simulink model "Simulation"  (R2023b)
settings: Solver=VariableStepAuto  StartTime=0.0  StopTime=20  RelTol=1e-3
undefined symbols (not defined in the file or in its folder): A, B, C, D, data
libraries: SignalEditorBlockLib x1
settings Model: Creator=ematric  LastModifiedBy=ematric

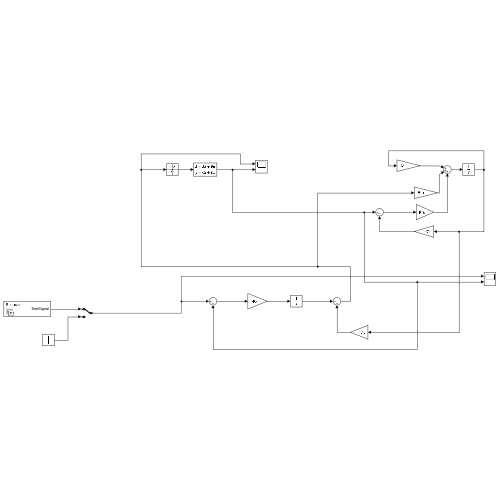
[thumbnail: Simulink's stored preview of the top-level diagram]
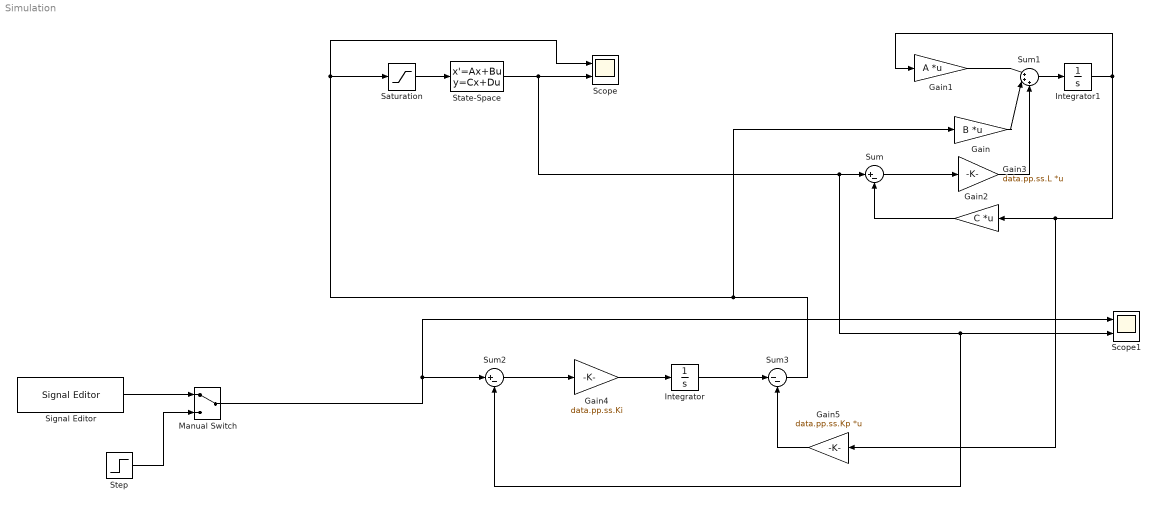
== system Simulation ==
  Gain : Gain  Gain=B  Multiplication=Matrix(K*u)
  Gain1 : Gain  Gain=A  Multiplication=Matrix(K*u)
  Gain2 : Gain  Gain=C  Multiplication=Matrix(K*u)
  Gain3 : Gain  Gain=data.pp.ss.L  Multiplication=Matrix(K*u)
  Gain4 : Gain  Gain=data.pp.ss.Ki
  Gain5 : Gain  Gain=data.pp.ss.Kp  Multiplication=Matrix(K*u)
  Integrator : Integrator
  Integrator1 : Integrator
  Manual Switch : ManualSwitch
  Saturation : Saturate  UpperLimit=5  LowerLimit=-5
  Scope : Scope  NumInputPorts=2
  Scope1 : Scope  NumInputPorts=2
  Signal Editor : SignalEditorBlockLib/Signal Editor  FileName=trajectories.mat  ActiveScenario=Scenario  ActiveSignal=TestSignal  IsBus=off  OutputBusObjectStr=Bus: BusObject  SampleTime=0  Interpolate=off  ZeroCross=off  OutputAfterFinalValue=Setting to zero  Unit=inherit  PreserveSignalName=on  ApplySigPropsToAllScenarios=on  ApplySigPropsToAllSignals=off
  State-Space : StateSpace  A=A  B=B  C=C  D=D  InitialCondition=0
  Step : Step  SampleTime=0
  Sum : Sum  Inputs=|+-
  Sum1 : Sum  Inputs=|+++
  Sum2 : Sum  Inputs=|+-
  Sum3 : Sum  Inputs=|--
  wires:
  Sum3/1 -> Gain/1, Scope/1, Saturation/1
  State-Space/1 -> Scope1/2, Sum2/2, Sum/1, Scope/2
  Step/1 -> Manual Switch/2
  Gain2/1 -> Sum/2
  Gain3/1 -> Sum1/3
  Gain/1 -> Sum1/2
  Sum/1 -> Gain3/1
  Sum1/1 -> Integrator1/1
  Gain1/1 -> Sum1/1
  Integrator1/1 -> Gain2/1, Gain5/1, Gain1/1
  Sum2/1 -> Gain4/1
  Gain4/1 -> Integrator/1
  Integrator/1 -> Sum3/1
  Manual Switch/1 -> Scope1/1, Sum2/1
  Gain5/1 -> Sum3/2
  Signal Editor/1 -> Manual Switch/1
  Saturation/1 -> State-Space/1
